simulink model "trial"  (R2021a)
settings: Solver=ode4  StartTime=0.0  StopTime=10  RelTol=1e-3
undefined symbols (not defined in the file): J, Rs
settings Model: Creator=Aashish Kalra  LastModifiedBy=Aashish Kalra

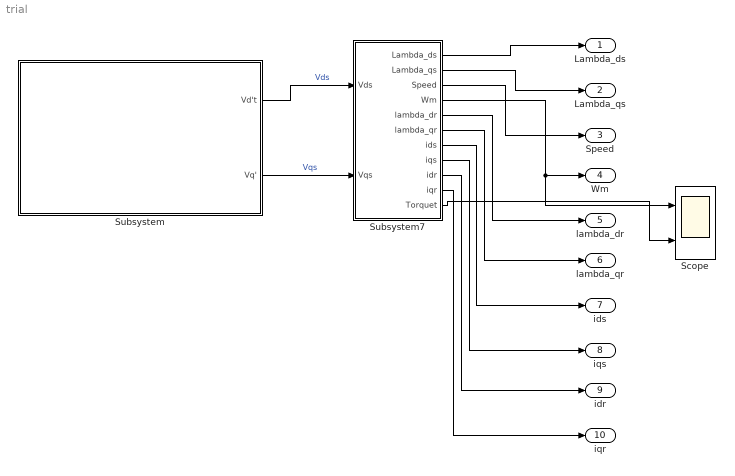
== system trial ==
  Scope : Scope  NumInputPorts=2
  Subsystem : Subsystem
  Subsystem7 : Subsystem
  Lambda_ds : Outport
  Lambda_qs : Outport  Port=2
  Speed : Outport  Port=3
  Wm : Outport  Port=4
  lambda_dr : Outport  Port=5
  lambda_qr : Outport  Port=6
  ids : Outport  Port=7
  iqs : Outport  Port=8
  idr : Outport  Port=9
  iqr : Outport  Port=10
  wires:
  Subsystem7/5(lambda_dr) -> lambda_dr/1
  Subsystem7/10(iqr) -> iqr/1
  Subsystem7/4(Wm) -> Scope/1, Wm/1
  Subsystem7/9(idr) -> idr/1
  Subsystem7/3(Speed) -> Speed/1
  Subsystem7/6(lambda_qr) -> lambda_qr/1
  Subsystem7/8(iqs) -> iqs/1
  Subsystem7/7(ids) -> ids/1
  Subsystem7/2(Lambda_qs) -> Lambda_qs/1
  Subsystem7/1(Lambda_ds) -> Lambda_ds/1
  Subsystem/2(Vq') -> Subsystem7/2(Vqs)  "Vqs"
  Subsystem/1(Vd't) -> Subsystem7/1(Vds)  "Vds"
  Subsystem7/11(Torquet) -> Scope/2

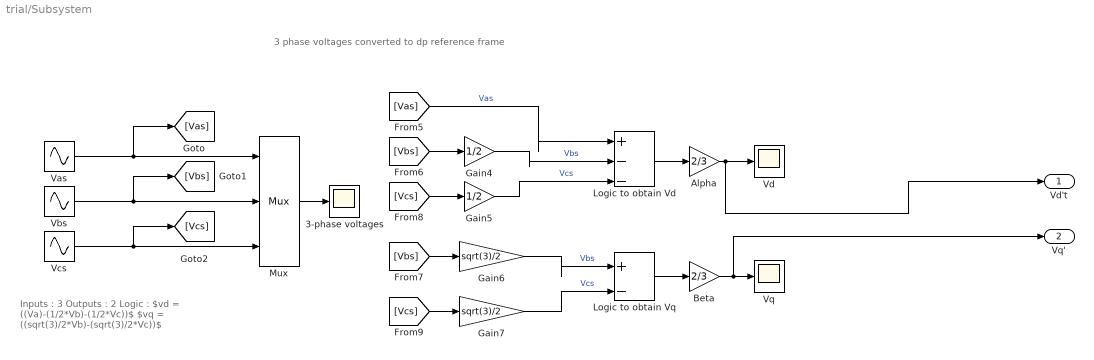
== system trial/Subsystem ==
  note: Inputs : 3
      | Outputs : 2
      |
      | Logic :
      | $vd = ((Va)-(1/2*Vb)-(1/2*Vc))$
      | $vq = ((sqrt(3)/2*Vb)-(sqrt(3)/2*Vc))$
  note: 3 phase voltages converted to dp reference frame
  3-phase voltages : Scope
  Alpha : Gain  Gain=2/3
  Beta : Gain  Gain=2/3
  Gain4 : Gain  Gain=1/2
  Gain5 : Gain  Gain=1/2
  Gain6 : Gain  Gain=sqrt(3)/2
  Gain7 : Gain  Gain=sqrt(3)/2
  Logic to obtain Vd : Sum  Inputs=|+--
  Logic to obtain Vq : Sum  Inputs=|+-
  Mux : Mux  Inputs=3
  Vas : Sin  Amplitude=220*sqrt(2)  Frequency=2*pi*60  Phase=(pi/2)  SampleTime=0
  Vbs : Sin  Amplitude=220*sqrt(2)  Frequency=2*pi*60  Phase=((-2*pi)/3)+(pi/2)  SampleTime=0
  Vcs : Sin  Amplitude=220*sqrt(2)  Frequency=2*pi*60  Phase=((2*pi)/3)+(pi/2)  SampleTime=0
  Vd : Scope
  Vq : Scope
  Vd't : Outport
  Vq' : Outport  Port=2
  wires:
  [Vbs] -> Gain4/1
  Vas/1 -> [Vas], Mux/1
  Beta/1 -> Vq'/1, Vq/1
  Vbs/1 -> [Vbs], Mux/2
  Mux/1 -> 3-phase voltages/1
  Vcs/1 -> [Vcs], Mux/3
  Gain5/1 -> Logic to obtain Vd/3  "Vcs"
  Logic to obtain Vq/1 -> Beta/1
  Gain6/1 -> Logic to obtain Vq/1  "Vbs"
  [Vbs] -> Gain6/1
  [Vas] -> Logic to obtain Vd/1  "Vas"
  [Vcs] -> Gain5/1
  Gain7/1 -> Logic to obtain Vq/2  "Vcs"
  Logic to obtain Vd/1 -> Alpha/1
  [Vcs] -> Gain7/1
  Gain4/1 -> Logic to obtain Vd/2  "Vbs"
  Alpha/1 -> Vd't/1, Vd/1

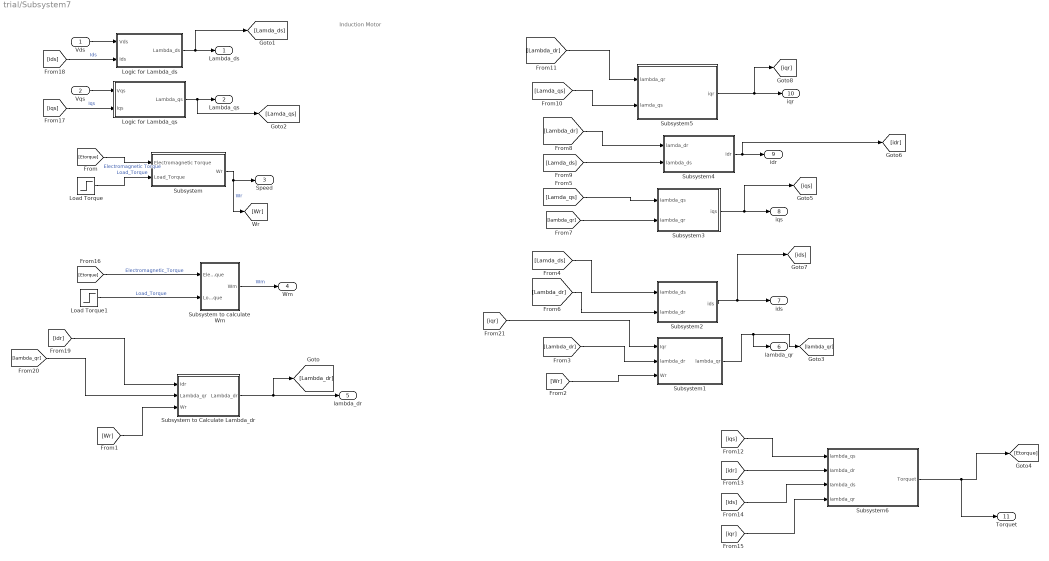
== system trial/Subsystem7 ==
  note: Induction Motor
  Vds : Inport
  Vqs : Inport  Port=2
  Load Torque : Step  Time=5  After=20  SampleTime=0
  Load Torque1 : Step  Time=5  After=20  SampleTime=0
  Logic for Lambda_ds : Subsystem
  Logic for Lambda_qs : Subsystem
  Subsystem : Subsystem
  Subsystem to Calculate Lambda_dr : Subsystem
  Subsystem to calculate Wm : Subsystem
  Subsystem1 : Subsystem
  Subsystem2 : Subsystem
  Subsystem3 : Subsystem
  Subsystem4 : Subsystem
  Subsystem5 : Subsystem
  Subsystem6 : Subsystem
  Lambda_ds : Outport
  Lambda_qs : Outport  Port=2
  Speed : Outport  Port=3
  Wm : Outport  Port=4
  lambda_dr : Outport  Port=5
  lambda_qr : Outport  Port=6
  ids : Outport  Port=7
  iqs : Outport  Port=8
  idr : Outport  Port=9
  iqr : Outport  Port=10
  Torquet : Outport  Port=11
  wires:
  Vqs/1 -> Logic for Lambda_qs/1(Vqs)
  Subsystem3/1(iqs) -> iqs/1, [iqs]
  [ids] -> Logic for Lambda_ds/2(Ids)  "Ids"
  [Wr] -> Subsystem to Calculate Lambda_dr/3(Wr)
  Subsystem to calculate Wm/1(Wm) -> Wm/1  "Wm"
  [Lambda_dr] -> Subsystem4/1(lamda_dr)
  Subsystem1/1(lambda_qr) -> lambda_qr/1, [lambda_qr]
  Subsystem2/1(ids) -> ids/1, [ids]
  [Etorque] -> Subsystem to calculate Wm/1(Electromagnetic_Torque)  "Electromagnetic_Torque"
  Subsystem4/1(idr) -> idr/1, [idr]
  [iqr] -> Subsystem1/1(Iqr)
  [Wr] -> Subsystem1/3(Wr)
  [iqs] -> Logic for Lambda_qs/2(Iqs)  "Iqs"
  Subsystem/1(Wr) -> Speed/1, [Wr]  "Wr"
  [iqr] -> Subsystem6/4(Iambda_qr)
  Logic for Lambda_qs/1(Lambda_qs) -> Lambda_qs/1, [Lamda_qs]
  [Lamda_ds] -> Subsystem2/1(Iambda_ds)
  [iqs] -> Subsystem6/1(lambda_qs)
  Load Torque/1 -> Subsystem/2(Load_Torque)  "Load_Torque"
  [Etorque] -> Subsystem/1(Electromagnetic Torque)  "Electromagnetic Torque"
  [ids] -> Subsystem6/3(Iambda_ds)
  [Lambda_dr] -> Subsystem5/1(lambda_qr)
  [idr] -> Subsystem to Calculate Lambda_dr/1(Idr)
  Vds/1 -> Logic for Lambda_ds/1(Vds)
  Subsystem to Calculate Lambda_dr/1(Lambda_dr) -> lambda_dr/1, [Lambda_dr]
  Subsystem5/1(iqr) -> iqr/1, [iqr]
  [lambda_qr] -> Subsystem3/2(Iambda_qr)
  [Lamda_qs] -> Subsystem3/1(Iambda_qs)
  Logic for Lambda_ds/1(Lambda_ds) -> Lambda_ds/1, [Lamda_ds]
  [lambda_qr] -> Subsystem to Calculate Lambda_dr/2(Lambda_qr)
  [Lambda_dr] -> Subsystem2/2(lambda_dr)
  Load Torque1/1 -> Subsystem to calculate Wm/2(Load_Torque)  "Load_Torque"
  [Lamda_ds] -> Subsystem4/2(lambda_ds)
  [Lambda_dr] -> Subsystem1/2(lambda_dr)
  [Lamda_qs] -> Subsystem5/2(lamda_qs)
  Subsystem6/1(Torquet) -> Torquet/1, [Etorque]
  [idr] -> Subsystem6/2(Iambda_dr)

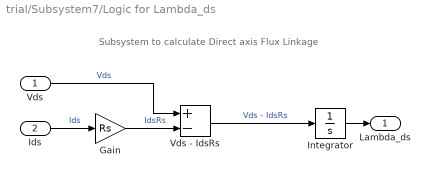
== system trial/Subsystem7/Logic for Lambda_ds ==
  note: Subsystem to calculate Direct axis Flux Linkage
  Vds : Inport
  Ids : Inport  Port=2
  Gain : Gain  Gain=Rs
  Integrator : Integrator
  Vds - IdsRs : Sum  Inputs=+-
  Lambda_ds : Outport
  wires:
  Ids/1 -> Gain/1  "Ids"
  Integrator/1 -> Lambda_ds/1
  Vds - IdsRs/1 -> Integrator/1  "Vds - IdsRs"
  Gain/1 -> Vds - IdsRs/2  "IdsRs"
  Vds/1 -> Vds - IdsRs/1  "Vds"

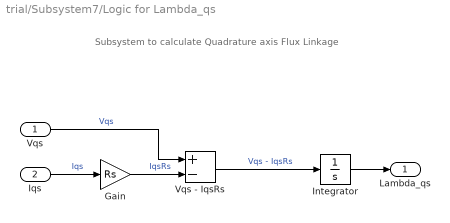
== system trial/Subsystem7/Logic for Lambda_qs ==
  note: Subsystem to calculate Quadrature axis Flux Linkage
  Vqs : Inport
  Iqs : Inport  Port=2
  Gain : Gain  Gain=Rs
  Integrator : Integrator
  Vqs - IqsRs : Sum  Inputs=+-
  Lambda_qs : Outport
  wires:
  Integrator/1 -> Lambda_qs/1
  Gain/1 -> Vqs - IqsRs/2  "IqsRs"
  Vqs - IqsRs/1 -> Integrator/1  "Vqs - IqsRs"
  Vqs/1 -> Vqs - IqsRs/1  "Vqs"
  Iqs/1 -> Gain/1  "Iqs"

== system trial/Subsystem7/Subsystem ==
  Electromagnetic Torque : Inport
  Load_Torque : Inport  Port=2
  (Te - Tl) : Sum  Inputs=+-
  Gain1 : Gain  Gain=44.9438
  Integrator4 : Integrator
  Wr : Outport
  wires:
  Load_Torque/1 -> (Te - Tl)/2
  Integrator4/1 -> Gain1/1
  (Te - Tl)/1 -> Integrator4/1
  Gain1/1 -> Wr/1  "Wr"
  Electromagnetic Torque/1 -> (Te - Tl)/1

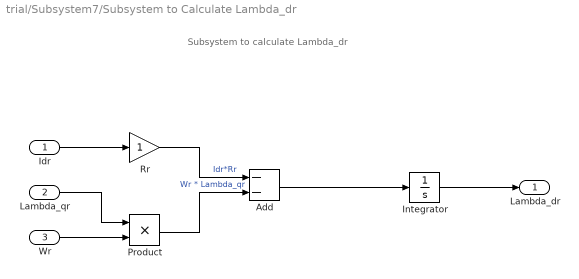
== system trial/Subsystem7/Subsystem to Calculate Lambda_dr ==
  note: Subsystem to calculate Lambda_dr
  Idr : Inport
  Lambda_qr : Inport  Port=2
  Wr : Inport  Port=3
  Add : Sum  Inputs=--
  Integrator : Integrator
  Product : Product
  Rr : Gain
  Lambda_dr : Outport
  wires:
  Add/1 -> Integrator/1
  Integrator/1 -> Lambda_dr/1
  Wr/1 -> Product/2
  Product/1 -> Add/2  "Wr * Lambda_qr"
  Lambda_qr/1 -> Product/1
  Idr/1 -> Rr/1
  Rr/1 -> Add/1  "Idr*Rr"

== system trial/Subsystem7/Subsystem to calculate Wm ==
  note: Subsytem to calculate Mechanical Speed
  Electromagnetic_Torque : Inport
  Load_Torque : Inport  Port=2
  (Te - Tl) : Sum  Inputs=+-
  Gain1 : Gain  Gain=1/J
  Integrator4 : Integrator
  Wm : Outport
  wires:
  Gain1/1 -> Integrator4/1
  Load_Torque/1 -> (Te - Tl)/2  "Load_Torque"
  Integrator4/1 -> Wm/1  "Wm"
  Electromagnetic_Torque/1 -> (Te - Tl)/1  "Electromagnetic_Torque"
  (Te - Tl)/1 -> Gain1/1

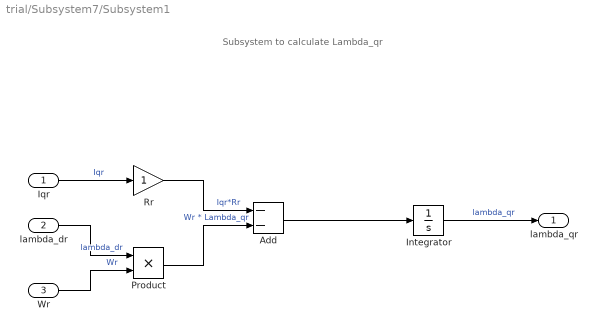
== system trial/Subsystem7/Subsystem1 ==
  note: Subsystem to calculate Lambda_qr
  Iqr : Inport
  lambda_dr : Inport  Port=2
  Wr : Inport  Port=3
  Add : Sum  Inputs=--
  Integrator : Integrator
  Product : Product
  Rr : Gain
  lambda_qr : Outport
  wires:
  Rr/1 -> Add/1  "Iqr*Rr"
  Product/1 -> Add/2  "Wr * Lambda_qr"
  Add/1 -> Integrator/1
  Integrator/1 -> lambda_qr/1  "lambda_qr"
  Iqr/1 -> Rr/1  "Iqr"
  Wr/1 -> Product/2  "Wr"
  lambda_dr/1 -> Product/1  "lambda_dr"

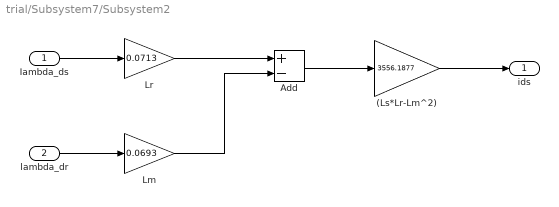
== system trial/Subsystem7/Subsystem2 ==
  Iambda_ds : Inport
  lambda_dr : Inport  Port=2
  (Ls*Lr-Lm^2) : Gain  Gain=3556.1877
  Add : Sum  Inputs=+-
  Lm : Gain  Gain=0.0693
  Lr : Gain  Gain=0.0713
  ids : Outport
  wires:
  (Ls*Lr-Lm^2)/1 -> ids/1
  Iambda_ds/1 -> Lr/1
  Lm/1 -> Add/2
  Add/1 -> (Ls*Lr-Lm^2)/1
  Lr/1 -> Add/1
  lambda_dr/1 -> Lm/1

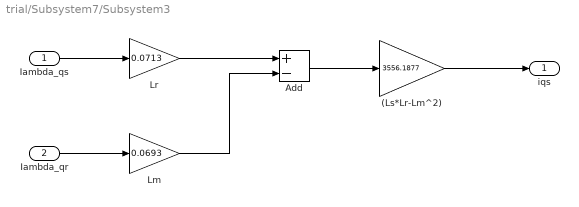
== system trial/Subsystem7/Subsystem3 ==
  Iambda_qs : Inport
  Iambda_qr : Inport  Port=2
  (Ls*Lr-Lm^2) : Gain  Gain=3556.1877
  Add : Sum  Inputs=+-
  Lm : Gain  Gain=0.0693
  Lr : Gain  Gain=0.0713
  iqs : Outport
  wires:
  Lr/1 -> Add/1
  Add/1 -> (Ls*Lr-Lm^2)/1
  (Ls*Lr-Lm^2)/1 -> iqs/1
  Lm/1 -> Add/2
  Iambda_qs/1 -> Lr/1
  Iambda_qr/1 -> Lm/1

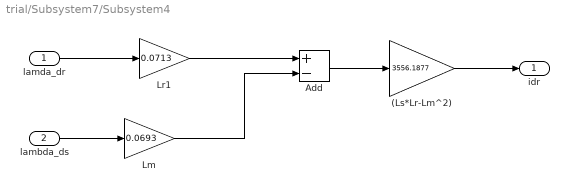
== system trial/Subsystem7/Subsystem4 ==
  lamda_dr : Inport
  lambda_ds : Inport  Port=2
  (Ls*Lr-Lm^2) : Gain  Gain=3556.1877
  Add : Sum  Inputs=+-
  Lm : Gain  Gain=0.0693
  Lr1 : Gain  Gain=0.0713
  idr : Outport
  wires:
  Lr1/1 -> Add/1
  Add/1 -> (Ls*Lr-Lm^2)/1
  (Ls*Lr-Lm^2)/1 -> idr/1
  lamda_dr/1 -> Lr1/1
  Lm/1 -> Add/2
  lambda_ds/1 -> Lm/1

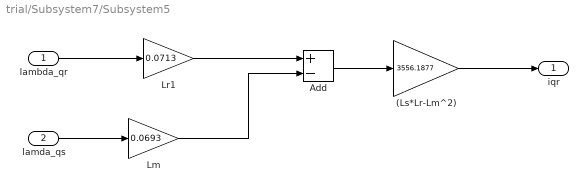
== system trial/Subsystem7/Subsystem5 ==
  lambda_qr : Inport
  lamda_qs : Inport  Port=2
  (Ls*Lr-Lm^2) : Gain  Gain=3556.1877
  Add : Sum  Inputs=+-
  Lm : Gain  Gain=0.0693
  Lr1 : Gain  Gain=0.0713
  iqr : Outport
  wires:
  Lm/1 -> Add/2
  Lr1/1 -> Add/1
  (Ls*Lr-Lm^2)/1 -> iqr/1
  Add/1 -> (Ls*Lr-Lm^2)/1
  lambda_qr/1 -> Lr1/1
  lamda_qs/1 -> Lm/1

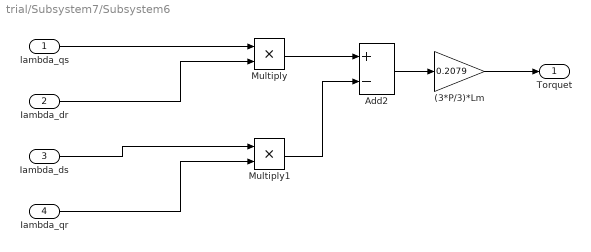
== system trial/Subsystem7/Subsystem6 ==
  lambda_qs : Inport
  Iambda_dr : Inport  Port=2
  Iambda_ds : Inport  Port=3
  Iambda_qr : Inport  Port=4
  (3*P/3)*Lm : Gain  Gain=0.2079
  Add2 : Sum  Inputs=+-
  Multiply : Product
  Multiply1 : Product
  Torquet : Outport
  wires:
  lambda_qs/1 -> Multiply/1
  Add2/1 -> (3*P/3)*Lm/1
  Multiply/1 -> Add2/1
  Iambda_qr/1 -> Multiply1/2
  Iambda_ds/1 -> Multiply1/1
  Multiply1/1 -> Add2/2
  (3*P/3)*Lm/1 -> Torquet/1
  Iambda_dr/1 -> Multiply/2
